simulink model "Third1"  (R2017b)
settings: Solver=VariableStepAuto  StartTime=0.0  StopTime=10.0  RelTol=1e-3
settings Model: Creator=17863  LastModifiedBy=17863

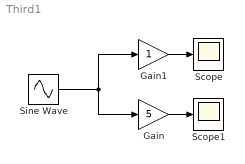
== system Third1 ==
  Gain : Gain  Gain=5
  Gain1 : Gain
  Scope : Scope
  Scope1 : Scope
  Sine Wave : Sin  Frequency=pi  SampleTime=0
  wires:
  Sine Wave/1 -> Gain/1, Gain1/1
  Gain1/1 -> Scope/1
  Gain/1 -> Scope1/1
